simulink model "sampleModel186"  (Simulink 9.1)
settings: Solver=VariableStepAuto  StartTime=0.0  StopTime=10.0  RelTol=1e-3
undefined symbols (not defined in the file): DiscIntNeverNeededParam, Newton, Raphson
libraries: simulink x39
(part 2 of 2)

== system sampleModel186/cfblk148/cfblk6 ==
  cfblk1 : Inport
  cfblk2 : Outport
  wires:
  cfblk1/1 -> cfblk2/1

== system sampleModel186/cfblk148/cfblk7 ==
  cfblk1 : Inport
  cfblk2 : Outport
  wires:
  cfblk1/1 -> cfblk2/1

== system sampleModel186/cfblk148/cfblk8 ==
  cfblk1 : Inport
  cfblk2 : Outport
  wires:
  cfblk1/1 -> cfblk2/1

== system sampleModel186/cfblk149/cfblk9 ==
  cfblk1 : Inport
  cfblk2 : Outport
  wires:
  cfblk1/1 -> cfblk2/1

== system sampleModel186/cfblk150/cfblk10 ==
  cfblk1 : Inport
  cfblk2 : Outport
  wires:
  cfblk1/1 -> cfblk2/1

== system sampleModel186/cfblk150/cfblk11 ==
  cfblk1 : Inport
  cfblk2 : Outport
  wires:
  cfblk1/1 -> cfblk2/1

== system sampleModel186/cfblk150/cfblk12 ==
  cfblk1 : Inport
  cfblk2 : Outport
  wires:
  cfblk1/1 -> cfblk2/1

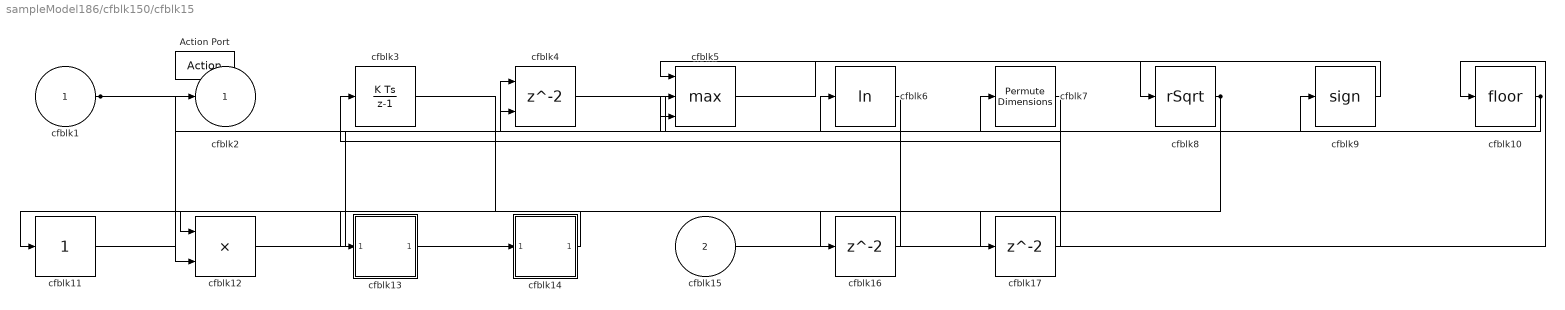
== system sampleModel186/cfblk150/cfblk15 ==
  cfblk1 : Inport
  cfblk15 : Inport  Port=2
  Action Port : ActionPort  ActionType=then
  cfblk10 : Rounding
  cfblk11 : simulink/Math Operations/Slider Gain  gain=1  low=0  high=2
  cfblk12 : Product  Inputs=**
  cfblk13 : Subsystem
  cfblk14 : Subsystem
  cfblk16 : Delay
  cfblk17 : Delay
  cfblk3 : DiscreteIntegrator  SampleTime=-1  ICPrevOutput=DiscIntNeverNeededParam  ICPrevScaledInput=DiscIntNeverNeededParam
  cfblk4 : Delay  ShowEnablePort=on
      settings: InputPortMap=u0,e6
  cfblk5 : MinMax  Function=max  Inputs=3
  cfblk6 : Math  Operator=log  SaturateOnIntegerOverflow=on
  cfblk7 : PermuteDimensions
  cfblk8 : Sqrt  Operator=rSqrt  AlgorithmType=Newton-Raphson  SaturateOnIntegerOverflow=on
  cfblk9 : Signum
  cfblk2 : Outport
  wires:
  cfblk9/1 -> cfblk5/1
  cfblk4/1 -> cfblk6/1
  cfblk5/1 -> cfblk8/1
  cfblk7/1 -> cfblk3/1
  cfblk14/1(cfblk2) -> cfblk11/1
  cfblk6/1 -> cfblk12/2
  cfblk11/1 -> cfblk7/1
  cfblk12/1 -> cfblk5/2
  cfblk13/1(cfblk2) -> cfblk14/1(cfblk1)
  cfblk10/1 -> cfblk9/1, cfblk4/2
  cfblk15/1 -> cfblk10/1
  cfblk8/1 -> cfblk13/1(cfblk1), cfblk17/1
  cfblk1/1 -> cfblk2/1, cfblk4/1
  cfblk3/1 -> cfblk16/1
  cfblk16/1 -> cfblk12/1
  cfblk17/1 -> cfblk5/3

== system sampleModel186/cfblk150/cfblk16 ==
  cfblk1 : Inport
  cfblk10 : Inport  Port=2
  Action Port : ActionPort  ActionType=else
  cfblk13 : Delay
  cfblk3 : DiscreteIntegrator  SampleTime=-1  ICPrevOutput=DiscIntNeverNeededParam  ICPrevScaledInput=DiscIntNeverNeededParam
  cfblk4 : Math  Operator=rem  SaturateOnIntegerOverflow=on
  cfblk5 : Bias  Bias=[286929198.710473]
  cfblk6 : Reshape
  cfblk7 : Constant  Value=[678656412.126638]  SampleTime=1
  cfblk8 : Subsystem
  cfblk9 : Subsystem
  cfblk2 : Outport
  cfblk11 : Outport  Port=2
  cfblk12 : Outport  Port=3
  wires:
  cfblk5/1 -> cfblk11/1
  cfblk4/1 -> cfblk5/1
  cfblk6/1 -> cfblk2/1
  cfblk1/1 -> cfblk4/1
  cfblk7/1 -> cfblk3/1
  cfblk10/1 -> cfblk12/1
  cfblk3/1 -> cfblk4/2, cfblk6/1
  cfblk8/1(cfblk2) -> cfblk9/1(cfblk1)
  cfblk9/1(cfblk2) -> cfblk13/1
  cfblk13/1 -> cfblk8/1(cfblk1)

== system sampleModel186/cfblk150/cfblk9 ==
  cfblk1 : Inport
  cfblk2 : Outport
  wires:
  cfblk1/1 -> cfblk2/1

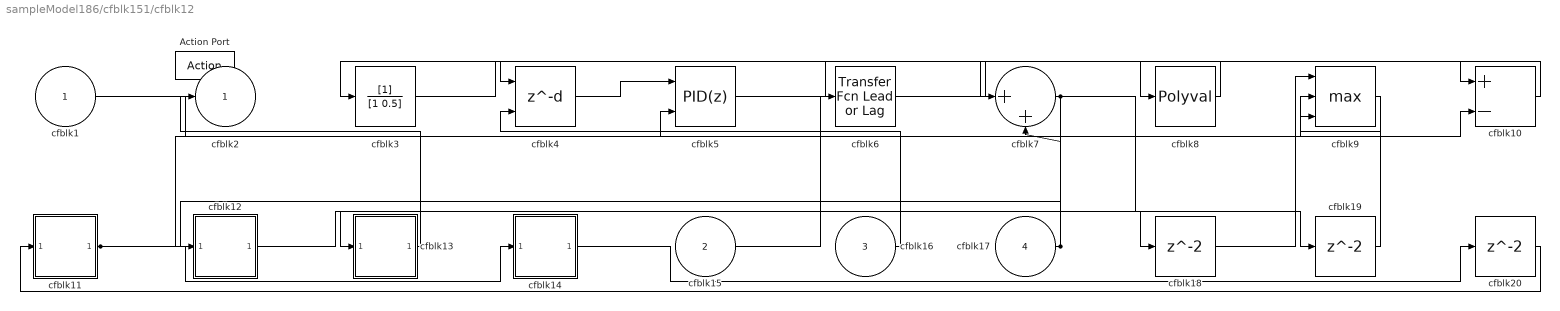
== system sampleModel186/cfblk151/cfblk12 ==
  cfblk1 : Inport
  cfblk15 : Inport  Port=2
  cfblk16 : Inport  Port=3
  cfblk17 : Inport  Port=4
  Action Port : ActionPort  ActionType=then
  cfblk10 : Sum  Inputs=+-
  cfblk11 : Subsystem
  cfblk12 : Subsystem
  cfblk13 : Subsystem
  cfblk14 : Subsystem
  cfblk18 : Delay
  cfblk19 : Delay
  cfblk20 : Delay
  cfblk3 : DiscreteFilter
  cfblk4 : Delay  DelayLengthSource=Input port
      settings: InputPortMap=u0,p1
  cfblk5 : simulink/Continuous/PID Controller (2DOF)  Controller=PID  TimeDomain=Discrete-time  SampleTime=-1  IntegratorMethod=Forward Euler  FilterMethod=Forward Euler  Form=Parallel  UseFilter=on  ControllerParametersSource=internal  P=1  I=1  D=0  N=100  b=1  c=1  InitialConditionSource=internal  InitialConditionForIntegrator=0  InitialConditionForFilter=0  ExternalReset=none  LimitOutput=off  UpperSaturationLimit=inf  LowerSaturationLimit=-inf  LinearizeAsGain=off  AntiWindupMode=none  Kb=1  TrackingMode=off  Kt=1  PParamMin=[]  PParamMax=[]  IParamMin=[]  IParamMax=[]  DParamMin=[]  DParamMax=[]  NParamMin=[]  NParamMax=[]  bParamMin=[]  bParamMax=[]  cParamMin=[]  cParamMax=[]  KbParamMin=[]  KbParamMax=[]  KtParamMin=[]  KtParamMax=[]  POutMin=[]  POutMax=[]  IOutMin=[]  IOutMax=[]  DOutMin=[]  DOutMax=[]  NOutMin=[]  NOutMax=[]  bOutMin=[]  bOutMax=[]  cOutMin=[]  cOutMax=[]  KbOutMin=[]  KbOutMax=[]  KtOutMin=[]  KtOutMax=[]  IntegratorOutMin=[]  IntegratorOutMax=[]  FilterOutMin=[]  FilterOutMax=[]  SumOutMin=[]  SumOutMax=[]  Sum1OutMin=[]  Sum1OutMax=[]  Sum2OutMin=[]  Sum2OutMax=[]  Sum3OutMin=[]  Sum3OutMax=[]  SumI1OutMin=[]  SumI1OutMax=[]  SumI2OutMin=[]  SumI2OutMax=[]  SumI3OutMin=[]  SumI3OutMax=[]  SumDOutMin=[]  SumDOutMax=[]  SaturationOutMin=[]  SaturationOutMax=[]  IntegratorContinuousStateAttributes=''  IntegratorStateMustResolveToSignalObject=off  IntegratorRTWStateStorageClass=Auto  FilterContinuousStateAttributes=''  FilterStateMustResolveToSignalObject=off  FilterRTWStateStorageClass=Auto  DifferentiatorICPrevScaledInput=0  DifferentiatorOutMin=[]  DifferentiatorOutMax=[]  FilterDiffOutCoefMin=[]  FilterDiffOutCoefMax=[]  SumDenOutMin=[]  SumDenOutMax=[]  SumNumOutMin=[]  SumNumOutMax=[]  ReciprocalOutMin=[]  ReciprocalOutMax=[]  DivideOutMin=[]  DivideOutMax=[]  TunerSelectOption=Transfer Function Based (PID Tuner App)
  cfblk6 : simulink/Discrete/Transfer Fcn Lead or Lag  PoleZ=0.95  ZeroZ=0.75  ICPrevOutput=0.0  ICPrevInput=0.0  DoSatur=off
      settings: SourceProductName=Simulink  SourceProductBaseCode=SL
  cfblk7 : Sum  Inputs=|++
  cfblk8 : Polyval  Coefs=[ +2.081618890e-019, -1.441693666e-014, +4.719686976e-010, -8.536869453e-006, +1.621573104e-001, -8.087801117e+001 ]
  cfblk9 : MinMax  Function=max  Inputs=3
  cfblk2 : Outport
  wires:
  cfblk10/1 -> cfblk4/1
  cfblk17/1 -> cfblk13/1(cfblk1), cfblk7/2
  cfblk11/1(cfblk2) -> cfblk14/1(cfblk1), cfblk10/2
  cfblk7/1 -> cfblk12/1(cfblk1), cfblk19/1
  cfblk1/1 -> cfblk9/2
  cfblk8/1 -> cfblk3/1
  cfblk6/1 -> cfblk8/1
  cfblk16/1 -> cfblk4/2
  cfblk4/1 -> cfblk5/1
  cfblk13/1(cfblk2) -> cfblk2/1
  cfblk3/1 -> cfblk10/1
  cfblk9/1 -> cfblk5/2
  cfblk5/1 -> cfblk7/1
  cfblk15/1 -> cfblk6/1
  cfblk12/1(cfblk2) -> cfblk18/1
  cfblk18/1 -> cfblk9/1
  cfblk19/1 -> cfblk9/3
  cfblk14/1(cfblk2) -> cfblk20/1
  cfblk20/1 -> cfblk11/1(cfblk1)

== system sampleModel186/cfblk151/cfblk13 ==
  cfblk1 : Inport
  Action Port : ActionPort  ActionType=else
  cfblk10 : Delay
  cfblk3 : Delay  ShowEnablePort=on
      settings: InputPortMap=u0,e6
  cfblk4 : Delay
  cfblk5 : Squeeze
  cfblk6 : Product  Inputs=**
  cfblk7 : Subsystem
  cfblk8 : Subsystem
  cfblk9 : Delay
  cfblk2 : Outport
  wires:
  cfblk6/1 -> cfblk8/1(cfblk1), cfblk9/1
  cfblk7/1(cfblk2) -> cfblk5/1, cfblk2/1
  cfblk5/1 -> cfblk6/1
  cfblk1/1 -> cfblk4/1
  cfblk3/1 -> cfblk7/1(cfblk1)
  cfblk4/1 -> cfblk3/2
  cfblk9/1 -> cfblk3/1
  cfblk8/1(cfblk2) -> cfblk10/1
  cfblk10/1 -> cfblk6/2

== system sampleModel186/cfblk151/cfblk8 ==
  cfblk1 : Inport
  cfblk2 : Outport
  wires:
  cfblk1/1 -> cfblk2/1

== system sampleModel186/cfblk152/cfblk10 ==
  cfblk1 : Inport
  cfblk2 : Outport
  wires:
  cfblk1/1 -> cfblk2/1

== system sampleModel186/cfblk152/cfblk11 ==
  cfblk1 : Inport
  cfblk2 : Outport
  wires:
  cfblk1/1 -> cfblk2/1

== system sampleModel186/cfblk152/cfblk12 ==
  cfblk1 : Inport
  cfblk2 : Outport
  wires:
  cfblk1/1 -> cfblk2/1

== system sampleModel186/cfblk152/cfblk7 ==
  cfblk1 : Inport
  cfblk2 : Outport
  wires:
  cfblk1/1 -> cfblk2/1

== system sampleModel186/cfblk152/cfblk8 ==
  cfblk1 : Inport
  cfblk2 : Outport
  wires:
  cfblk1/1 -> cfblk2/1

== system sampleModel186/cfblk152/cfblk9 ==
  cfblk1 : Inport
  cfblk2 : Outport
  wires:
  cfblk1/1 -> cfblk2/1

== system sampleModel186/cfblk153/cfblk4 ==
  cfblk1 : Inport
  cfblk2 : Outport
  wires:
  cfblk1/1 -> cfblk2/1

== system sampleModel186/cfblk153/cfblk5 ==
  cfblk1 : Inport
  cfblk2 : Outport
  wires:
  cfblk1/1 -> cfblk2/1

== system sampleModel186/cfblk153/cfblk6 ==
  cfblk1 : Inport
  cfblk2 : Outport
  wires:
  cfblk1/1 -> cfblk2/1

== system sampleModel186/cfblk153/cfblk7 ==
  cfblk1 : Inport
  cfblk2 : Outport
  wires:
  cfblk1/1 -> cfblk2/1

== system sampleModel186/cfblk153/cfblk8 ==
  cfblk1 : Inport
  cfblk2 : Outport
  wires:
  cfblk1/1 -> cfblk2/1

== system sampleModel186/cfblk154/cfblk10 ==
  cfblk1 : Inport
  cfblk2 : Outport
  wires:
  cfblk1/1 -> cfblk2/1

== system sampleModel186/cfblk154/cfblk11 ==
  cfblk1 : Inport
  cfblk2 : Outport
  wires:
  cfblk1/1 -> cfblk2/1

== system sampleModel186/cfblk154/cfblk12 ==
  cfblk1 : Inport
  cfblk2 : Outport
  wires:
  cfblk1/1 -> cfblk2/1

== system sampleModel186/cfblk154/cfblk13 ==
  cfblk1 : Inport
  cfblk2 : Outport
  wires:
  cfblk1/1 -> cfblk2/1

== system sampleModel186/cfblk155/cfblk4 ==
  cfblk1 : Inport
  cfblk2 : Outport
  wires:
  cfblk1/1 -> cfblk2/1

== system sampleModel186/cfblk156/cfblk10 ==
  cfblk1 : Inport
  cfblk2 : Outport
  wires:
  cfblk1/1 -> cfblk2/1

== system sampleModel186/cfblk156/cfblk7 ==
  cfblk1 : Inport
  cfblk2 : Outport
  wires:
  cfblk1/1 -> cfblk2/1

== system sampleModel186/cfblk156/cfblk8 ==
  cfblk1 : Inport
  cfblk2 : Outport
  wires:
  cfblk1/1 -> cfblk2/1

== system sampleModel186/cfblk156/cfblk9 ==
  cfblk1 : Inport
  cfblk2 : Outport
  wires:
  cfblk1/1 -> cfblk2/1

== system sampleModel186/cfblk157/cfblk5 ==
  cfblk1 : Inport
  cfblk2 : Outport
  wires:
  cfblk1/1 -> cfblk2/1

== system sampleModel186/cfblk157/cfblk6 ==
  cfblk1 : Inport
  cfblk2 : Outport
  wires:
  cfblk1/1 -> cfblk2/1

== system sampleModel186/cfblk157/cfblk7 ==
  cfblk1 : Inport
  cfblk2 : Outport
  wires:
  cfblk1/1 -> cfblk2/1

== system sampleModel186/cfblk158/cfblk10 ==
  cfblk1 : Inport
  cfblk2 : Outport
  wires:
  cfblk1/1 -> cfblk2/1

== system sampleModel186/cfblk158/cfblk11 ==
  cfblk1 : Inport
  cfblk2 : Outport
  wires:
  cfblk1/1 -> cfblk2/1

== system sampleModel186/cfblk158/cfblk12 ==
  cfblk1 : Inport
  cfblk2 : Outport
  wires:
  cfblk1/1 -> cfblk2/1

== system sampleModel186/cfblk158/cfblk9 ==
  cfblk1 : Inport
  cfblk2 : Outport
  wires:
  cfblk1/1 -> cfblk2/1

== system sampleModel186/cfblk159/cfblk10 ==
  cfblk1 : Inport
  cfblk2 : Outport
  wires:
  cfblk1/1 -> cfblk2/1

== system sampleModel186/cfblk159/cfblk11 ==
  cfblk1 : Inport
  cfblk2 : Outport
  wires:
  cfblk1/1 -> cfblk2/1

== system sampleModel186/cfblk159/cfblk9 ==
  cfblk1 : Inport
  cfblk2 : Outport
  wires:
  cfblk1/1 -> cfblk2/1

== system sampleModel186/cfblk160/cfblk8 ==
  cfblk1 : Inport
  cfblk12 : Inport  Port=2
  Action Port : ActionPort  ActionType=then
  cfblk10 : Subsystem
  cfblk11 : Subsystem
  cfblk14 : Delay
  cfblk3 : UnitDelay  SampleTime=-1
  cfblk4 : Delay
  cfblk5 : Delay
  cfblk6 : Sum  Inputs=|++
  cfblk7 : Reshape
  cfblk8 : Constant  Value=[-104552540.702008]  SampleTime=1
  cfblk9 : Subsystem
  cfblk2 : Outport
  cfblk13 : Outport  Port=2
  wires:
  cfblk4/1 -> cfblk10/1(cfblk1)
  cfblk11/1(cfblk2) -> cfblk7/1
  cfblk9/1(cfblk2) -> cfblk11/1(cfblk1)
  cfblk3/1 -> cfblk5/1
  cfblk5/1 -> cfblk13/1
  cfblk6/1 -> cfblk9/1(cfblk1)
  cfblk7/1 -> cfblk2/1
  cfblk12/1 -> cfblk6/1
  cfblk8/1 -> cfblk3/1
  cfblk1/1 -> cfblk6/2
  cfblk10/1(cfblk2) -> cfblk14/1
  cfblk14/1 -> cfblk4/1

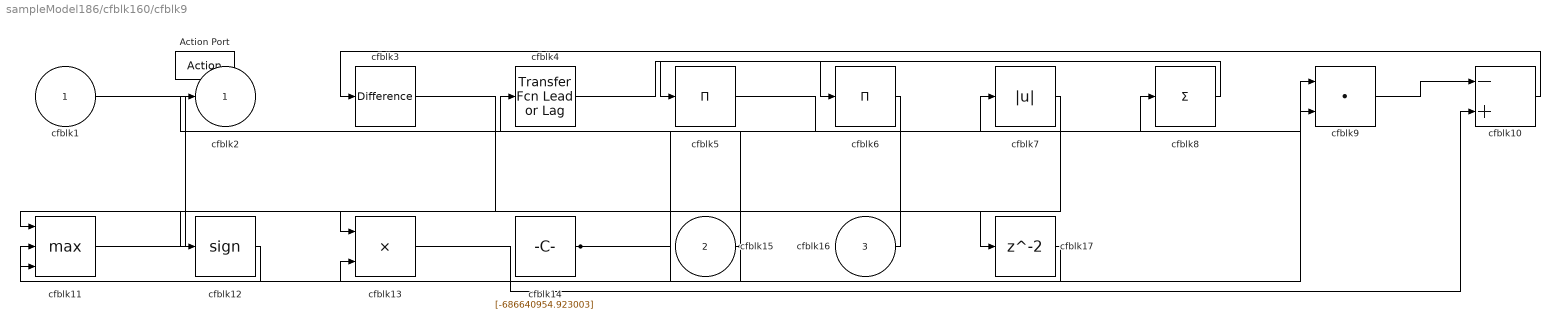
== system sampleModel186/cfblk160/cfblk9 ==
  cfblk1 : Inport
  cfblk15 : Inport  Port=2
  cfblk16 : Inport  Port=3
  Action Port : ActionPort  ActionType=else
  cfblk10 : Sum  Inputs=-+
  cfblk11 : MinMax  Function=max  Inputs=3
  cfblk12 : Signum
  cfblk13 : Product  Inputs=**
  cfblk14 : Constant  Value=[-686640954.923003]  SampleTime=1
  cfblk17 : Delay
  cfblk3 : simulink/Discrete/Difference  ICPrevInput=0.0  OutMin=[]  OutMax=[]  OutDataTypeStr=Inherit: Inherit via back propagation  OutDataType=fixdt(1, 16)  OutScaling=2^-10  DoSatur=off
  cfblk4 : simulink/Discrete/Transfer Fcn Lead or Lag  PoleZ=0.95  ZeroZ=0.75  ICPrevOutput=0.0  ICPrevInput=0.0  DoSatur=off
      settings: SourceProductName=Simulink  SourceProductBaseCode=SL
  cfblk5 : Product  Inputs=*
  cfblk6 : Product  Inputs=*
  cfblk7 : Abs
  cfblk8 : Sum  Inputs=+
  cfblk9 : DotProduct  InputSameDT=on  OutDataTypeStr=Inherit: Inherit via internal rule
  cfblk2 : Outport
  wires:
  cfblk1/1 -> cfblk7/1
  cfblk8/1 -> cfblk5/1
  cfblk11/1 -> cfblk4/1
  cfblk6/1 -> cfblk13/1
  cfblk14/1 -> cfblk9/1, cfblk8/1
  cfblk4/1 -> cfblk6/1
  cfblk7/1 -> cfblk11/1
  cfblk16/1 -> cfblk12/1
  cfblk9/1 -> cfblk10/1
  cfblk15/1 -> cfblk2/1, cfblk11/3
  cfblk5/1 -> cfblk9/2
  cfblk13/1 -> cfblk10/2
  cfblk12/1 -> cfblk11/2
  cfblk10/1 -> cfblk3/1
  cfblk3/1 -> cfblk17/1
  cfblk17/1 -> cfblk13/2

== system sampleModel186/cfblk161/cfblk10 ==
  cfblk1 : Inport
  cfblk2 : Outport
  wires:
  cfblk1/1 -> cfblk2/1

== system sampleModel186/cfblk161/cfblk11 ==
  cfblk1 : Inport
  cfblk2 : Outport
  wires:
  cfblk1/1 -> cfblk2/1

== system sampleModel186/cfblk161/cfblk17 ==
  cfblk1 : Inport
  cfblk9 : Inport  Port=2
  cfblk10 : Inport  Port=3
  cfblk11 : Inport  Port=4
  Action Port : ActionPort  ActionType=then
  cfblk3 : Product  Inputs=*
  cfblk4 : Squeeze
  cfblk5 : Bias  Bias=[280600987.660149]
  cfblk6 : Bias  Bias=[-755800568.597337]
  cfblk7 : ComplexToMagnitudeAngle
  cfblk8 : Subsystem
  cfblk2 : Outport
  wires:
  cfblk9/1 -> cfblk5/1
  cfblk6/1 -> cfblk2/1
  cfblk11/1 -> cfblk4/1
  cfblk1/1 -> cfblk7/1
  cfblk5/1 -> cfblk6/1
  cfblk8/1(cfblk2) -> cfblk3/1
  cfblk7/1 -> cfblk8/1(cfblk1)

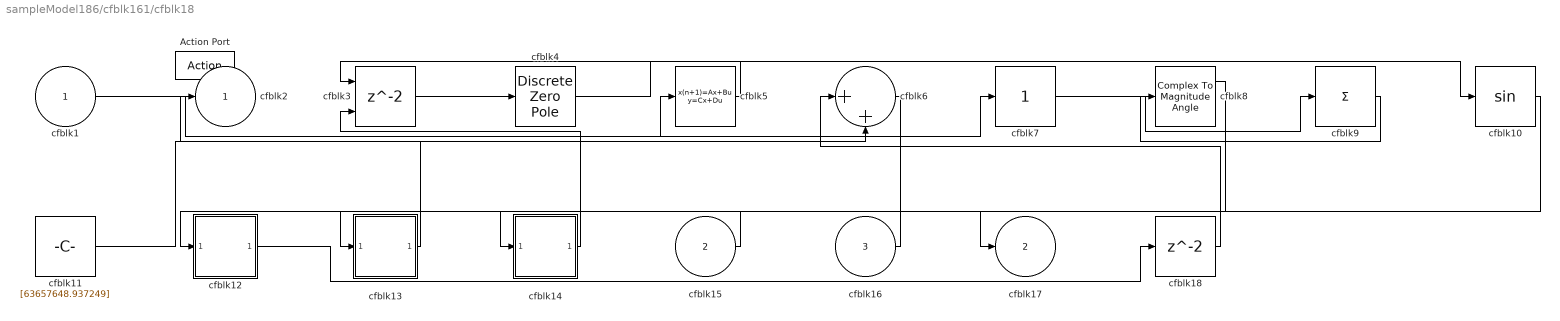
== system sampleModel186/cfblk161/cfblk18 ==
  cfblk1 : Inport
  cfblk15 : Inport  Port=2
  cfblk16 : Inport  Port=3
  Action Port : ActionPort  ActionType=else
  cfblk10 : Trigonometry
  cfblk11 : Constant  Value=[63657648.937249]  SampleTime=1
  cfblk12 : Subsystem
  cfblk13 : Subsystem
  cfblk14 : Subsystem
  cfblk18 : Delay
  cfblk3 : Delay  ShowEnablePort=on
      settings: InputPortMap=u0,e6
  cfblk4 : DiscreteZeroPole  Poles=[0 0.5]  Gain=1  SampleTime=-1
  cfblk5 : DiscreteStateSpace  SampleTime=-1
  cfblk6 : Sum  Inputs=|++
  cfblk7 : simulink/Math Operations/Slider Gain  gain=1  low=0  high=2
  cfblk8 : ComplexToMagnitudeAngle
  cfblk9 : Sum  Inputs=+
  cfblk2 : Outport
  cfblk17 : Outport  Port=2
  wires:
  cfblk16/1 -> cfblk5/1
  cfblk4/1 -> cfblk10/1
  cfblk7/1 -> cfblk9/1
  cfblk1/1 -> cfblk7/1
  cfblk10/1 -> cfblk17/1
  cfblk9/1 -> cfblk8/1
  cfblk13/1(cfblk2) -> cfblk2/1
  cfblk3/1 -> cfblk4/1
  cfblk15/1 -> cfblk14/1(cfblk1)
  cfblk6/1 -> cfblk12/1(cfblk1)
  cfblk11/1 -> cfblk6/2
  cfblk5/1 -> cfblk3/1
  cfblk14/1(cfblk2) -> cfblk3/2
  cfblk8/1 -> cfblk13/1(cfblk1)
  cfblk12/1(cfblk2) -> cfblk18/1
  cfblk18/1 -> cfblk6/1

== system sampleModel186/cfblk162/cfblk12 ==
  cfblk1 : Inport
  cfblk2 : Outport
  wires:
  cfblk1/1 -> cfblk2/1

== system sampleModel186/cfblk147/cfblk14/cfblk7 ==
  cfblk1 : Inport
  cfblk2 : Outport
  wires:
  cfblk1/1 -> cfblk2/1

== system sampleModel186/cfblk147/cfblk14/cfblk8 ==
  cfblk1 : Inport
  cfblk2 : Outport
  wires:
  cfblk1/1 -> cfblk2/1

== system sampleModel186/cfblk150/cfblk15/cfblk13 ==
  cfblk1 : Inport
  cfblk2 : Outport
  wires:
  cfblk1/1 -> cfblk2/1

== system sampleModel186/cfblk150/cfblk15/cfblk14 ==
  cfblk1 : Inport
  cfblk2 : Outport
  wires:
  cfblk1/1 -> cfblk2/1

== system sampleModel186/cfblk150/cfblk16/cfblk8 ==
  cfblk1 : Inport
  cfblk2 : Outport
  wires:
  cfblk1/1 -> cfblk2/1

== system sampleModel186/cfblk150/cfblk16/cfblk9 ==
  cfblk1 : Inport
  cfblk2 : Outport
  wires:
  cfblk1/1 -> cfblk2/1

== system sampleModel186/cfblk151/cfblk12/cfblk11 ==
  cfblk1 : Inport
  cfblk2 : Outport
  wires:
  cfblk1/1 -> cfblk2/1

== system sampleModel186/cfblk151/cfblk12/cfblk12 ==
  cfblk1 : Inport
  cfblk2 : Outport
  wires:
  cfblk1/1 -> cfblk2/1

== system sampleModel186/cfblk151/cfblk12/cfblk13 ==
  cfblk1 : Inport
  cfblk2 : Outport
  wires:
  cfblk1/1 -> cfblk2/1

== system sampleModel186/cfblk151/cfblk12/cfblk14 ==
  cfblk1 : Inport
  cfblk2 : Outport
  wires:
  cfblk1/1 -> cfblk2/1

== system sampleModel186/cfblk151/cfblk13/cfblk7 ==
  cfblk1 : Inport
  cfblk2 : Outport
  wires:
  cfblk1/1 -> cfblk2/1

== system sampleModel186/cfblk151/cfblk13/cfblk8 ==
  cfblk1 : Inport
  cfblk2 : Outport
  wires:
  cfblk1/1 -> cfblk2/1

== system sampleModel186/cfblk160/cfblk8/cfblk10 ==
  cfblk1 : Inport
  cfblk2 : Outport
  wires:
  cfblk1/1 -> cfblk2/1

== system sampleModel186/cfblk160/cfblk8/cfblk11 ==
  cfblk1 : Inport
  cfblk2 : Outport
  wires:
  cfblk1/1 -> cfblk2/1

== system sampleModel186/cfblk160/cfblk8/cfblk9 ==
  cfblk1 : Inport
  cfblk2 : Outport
  wires:
  cfblk1/1 -> cfblk2/1

== system sampleModel186/cfblk161/cfblk17/cfblk8 ==
  cfblk1 : Inport
  cfblk2 : Outport
  wires:
  cfblk1/1 -> cfblk2/1

== system sampleModel186/cfblk161/cfblk18/cfblk12 ==
  cfblk1 : Inport
  cfblk2 : Outport
  wires:
  cfblk1/1 -> cfblk2/1

== system sampleModel186/cfblk161/cfblk18/cfblk13 ==
  cfblk1 : Inport
  cfblk2 : Outport
  wires:
  cfblk1/1 -> cfblk2/1

== system sampleModel186/cfblk161/cfblk18/cfblk14 ==
  cfblk1 : Inport
  cfblk2 : Outport
  wires:
  cfblk1/1 -> cfblk2/1
